simulink model "Modelo_ideal"  (R2021a)
settings: Solver=VariableStepAuto  StartTime=0.0  StopTime=7  RelTol=1e-3
values from neighbouring files (symbols this model uses):
  alpha = 0.5    [Parametros.m]
  Cc = 1000    [Parametros.m]
  Cmax = 900    [Parametros.m]
  Cmin = 100    [Parametros.m]
  Kc = 16000    [Parametros.m]
  Kr = 160000    [Parametros.m]
  Mc = 250    [Parametros.m]
  Mr = 45    [Parametros.m]
undefined symbols (not defined in the file or in its folder): sigbuilder_block
settings Model: Creator=fhlla  LastModifiedBy=fhlla

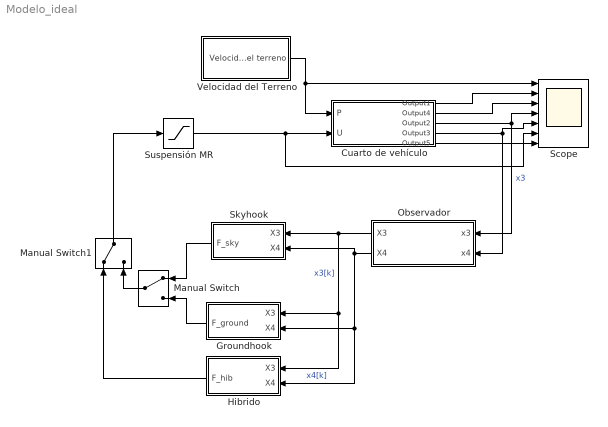
== system Modelo_ideal ==
  Cuarto de vehículo : Subsystem
  Groundhook : Subsystem
  Hibrido : Subsystem
  Manual Switch : ManualSwitch
  Manual Switch1 : ManualSwitch
  Observador : Subsystem
  Scope : Scope  NumInputPorts=7
  Skyhook : Subsystem
  Suspensión MR : Saturate  UpperLimit=10000  LowerLimit=-10000
  Velocidad del Terreno : Subsystem  Tag=STV Subsys  LoadFcn=sigbuilder_block('load');  StartFcn=sigbuilder_block('start');  StopFcn=sigbuilder_block('stop');  ClipboardFcn=sigbuilder_block('clipboard');  mask(Sigbuilder block){tuvar=[0:10]}
      mask help: Simulink:masks:SigbuilderBlock_MD
      mask init:
      | if ~strcmp(get_param(bdroot(gcbh),'SimulationStatus'),'stopped') tuvar = sigbuilder_block('maskInit'); end
      settings: CopyFcn=sigbuilder_block('copy');  DeleteFcn=sigbuilder_block('delete');  ModelCloseFcn=sigbuilder_block('modelClose');  PreSaveFcn=sigbuilder_block('preSave');  PauseFcn=sigbuilder_block('pause');  ContinueFcn=sigbuilder_block('continue');  NameChangeFcn=sigbuilder_block('namechange');  OpenFcn=sigbuilder_block('open',[0 30 1024.5 488.25 ]);  CloseFcn=sigbuilder_block('close');
      mask Display: plot(0, 0, 100, 100,[2, 2, 32, 32, 2], [68, 8, 8, 68, 68],[32, 2], [38, 38], [32, 19, 2],[53, 60, 44], [32, 17, 17, 2],[16, 16, 31, 31]);txt = getActiveGroup(gcbh);text(2, 100, txt,'verticalAlignment', 'top');
  wires:
  Suspensión MR/1 -> Cuarto de vehículo/2(U), Scope/6
  Velocidad del Terreno/1(Velocidad del terreno) -> Cuarto de vehículo/1(P), Scope/1
  Cuarto de vehículo/3(Output2) -> Observador/1(x3), Scope/4  "x3"
  Cuarto de vehículo/4(Output3) -> Observador/2(x4), Scope/5
  Skyhook/1(F_sky) -> Manual Switch/1
  Groundhook/1(F_ground) -> Manual Switch/2
  Cuarto de vehículo/1(Output1) -> Scope/2
  Cuarto de vehículo/2(Output4) -> Scope/3
  Observador/1(X3) -> Skyhook/1(X3), Hibrido/1(X3), Groundhook/1(X3)  "x3[k]"
  Observador/2(X4) -> Skyhook/2(X4), Hibrido/2(X4), Groundhook/2(X4)  "x4[k]"
  Manual Switch1/1 -> Suspensión MR/1
  Manual Switch/1 -> Manual Switch1/2
  Hibrido/1(F_hib) -> Manual Switch1/1
  Cuarto de vehículo/5(Output5) -> Scope/7

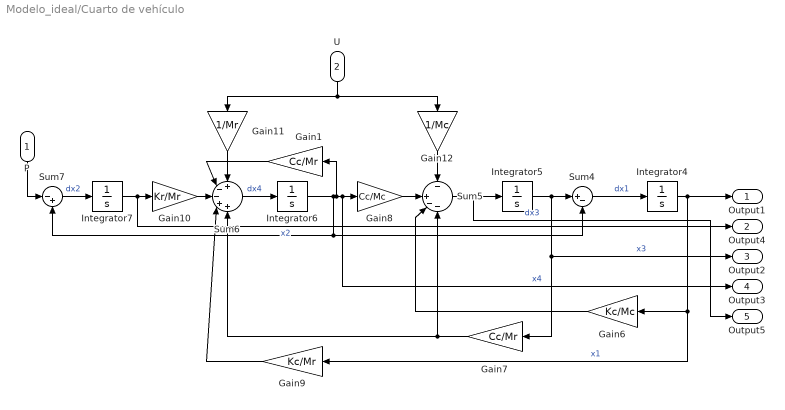
== system Modelo_ideal/Cuarto de vehículo ==
  P : Inport
  U : Inport  Port=2
  Gain1 : Gain  Gain=Cc/Mr
  Gain10 : Gain  Gain=Kr/Mr
  Gain11 : Gain  Gain=1/Mr
  Gain12 : Gain  Gain=1/Mc
  Gain6 : Gain  Gain=Kc/Mc
  Gain7 : Gain  Gain=Cc/Mr
  Gain8 : Gain  Gain=Cc/Mc
  Gain9 : Gain  Gain=Kc/Mr
  Integrator{4..7} (4 alike) : Integrator
  Sum4 : Sum  Inputs=|+-
  Sum5 : Sum  Inputs=-|+--
  Sum6 : Sum  Inputs=+--++
  Sum7 : Sum  Inputs=|-+
  Output1 : Outport
  Output4 : Outport  Port=2
  Output2 : Outport  Port=3
  Output3 : Outport  Port=4
  Output5 : Outport  Port=5
  wires:
  Gain6/1 -> Sum5/3
  Gain11/1 -> Sum6/1
  Gain8/1 -> Sum5/2
  Integrator5/1 -> Sum4/1, Output2/1, Gain7/1  "x3"
  Integrator7/1 -> Output4/1, Gain10/1  "x2"
  Integrator4/1 -> Gain9/1, Gain6/1, Output1/1  "x1"
  Gain10/1 -> Sum6/3
  Sum4/1 -> Integrator4/1  "dx1"
  Gain9/1 -> Sum6/4
  Gain7/1 -> Sum6/5, Sum5/4
  Sum5/1 -> Output5/1, Integrator5/1  "dx3"
  U/1 -> Gain12/1, Gain11/1
  Sum7/1 -> Integrator7/1  "dx2"
  P/1 -> Sum7/1
  Integrator6/1 -> Gain1/1, Output3/1, Gain8/1, Sum7/2, Sum4/2  "x4"
  Gain12/1 -> Sum5/1
  Sum6/1 -> Integrator6/1  "dx4"
  Gain1/1 -> Sum6/2

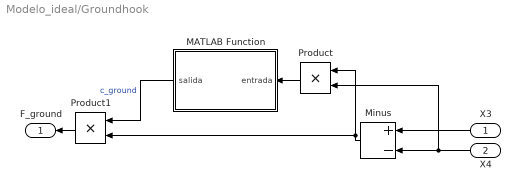
== system Modelo_ideal/Groundhook ==
  X3 : Inport
  X4 : Inport  Port=2
  MATLAB Function : MATLAB Function  TreatAsAtomicUnit=on
  Minus : Sum  Inputs=+-
  Product : Product
  Product1 : Product
  F_ground : Outport
  wires:
  Product/1 -> MATLAB Function/1(entrada)
  X4/1 -> Minus/2, Product/2
  Product1/1 -> F_ground/1
  Minus/1 -> Product1/2, Product/1
  MATLAB Function/1(salida) -> Product1/1  "c_ground"
  X3/1 -> Minus/1

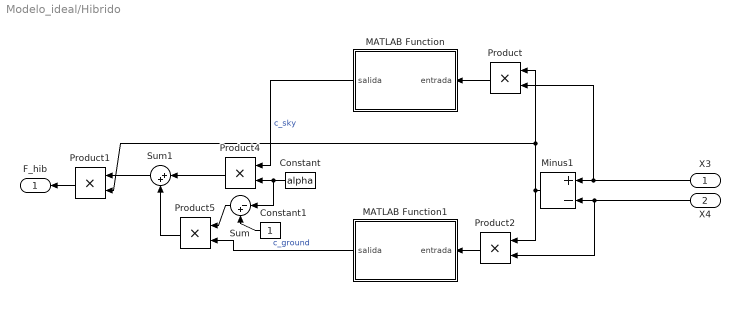
== system Modelo_ideal/Hibrido ==
  X3 : Inport
  X4 : Inport  Port=2
  Constant : Constant  Value=alpha
  Constant1 : Constant
  MATLAB Function : MATLAB Function  TreatAsAtomicUnit=on
  MATLAB Function1 : MATLAB Function  TreatAsAtomicUnit=on
  Minus1 : Sum  Inputs=+-
  Product{,1..2,4..5} (5 alike) : Product
  Sum : Sum  Inputs=|-+
  Sum1 : Sum  Inputs=|++
  F_hib : Outport
  wires:
  Product/1 -> MATLAB Function/1(entrada)
  MATLAB Function/1(salida) -> Product4/1  "c_sky"
  X3/1 -> Product/2, Minus1/1
  X4/1 -> Product2/2, Minus1/2
  Minus1/1 -> Product2/1, Product1/2, Product/1
  Product2/1 -> MATLAB Function1/1(entrada)
  MATLAB Function1/1(salida) -> Product5/2  "c_ground"
  Constant/1 -> Sum/1, Product4/2
  Constant1/1 -> Sum/2
  Sum/1 -> Product5/1
  Product5/1 -> Sum1/2
  Product4/1 -> Sum1/1
  Sum1/1 -> Product1/1
  Product1/1 -> F_hib/1

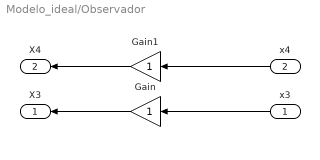
== system Modelo_ideal/Observador ==
  x3 : Inport
  x4 : Inport  Port=2
  Gain : Gain
  Gain1 : Gain
  X3 : Outport
  X4 : Outport  Port=2
  wires:
  x3/1 -> Gain/1
  x4/1 -> Gain1/1
  Gain/1 -> X3/1
  Gain1/1 -> X4/1

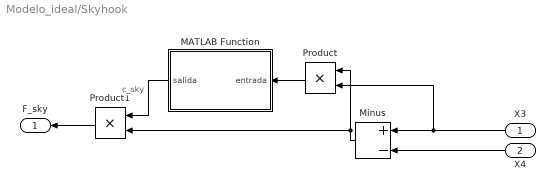
== system Modelo_ideal/Skyhook ==
  X3 : Inport
  X4 : Inport  Port=2
  MATLAB Function : MATLAB Function  TreatAsAtomicUnit=on
  Minus : Sum  Inputs=+-
  Product : Product
  Product1 : Product
  F_sky : Outport
  wires:
  Minus/1 -> Product1/2, Product/1
  Product/1 -> MATLAB Function/1(entrada)
  MATLAB Function/1(salida) -> Product1/1  "c_sky"
  Product1/1 -> F_sky/1
  X4/1 -> Minus/2
  X3/1 -> Product/2, Minus/1

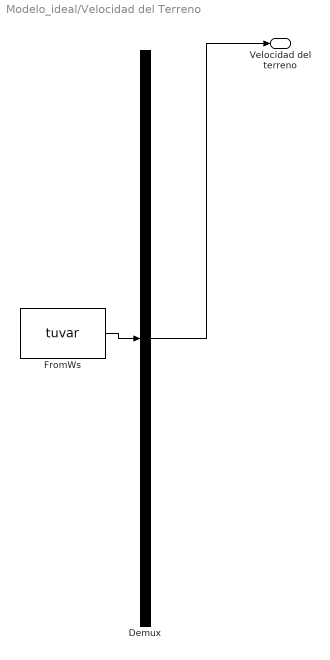
== system Modelo_ideal/Velocidad del Terreno ==
  Demux : Demux  Tag=STV Demux  Outputs=1
  FromWs : FromWorkspace  Tag=STV FromWs  VariableName=tuvar  SampleTime=0
      SigBuilderData=|
      | common.afterFinalStr = 'Extrapolate'
      | common.sampleTime = 0
      | dataSet.timeRange = [0 11.5]
      | dataSet.name = 'Group 1'
      | sbobj.Groups.Name = 'Group 1'
      | sbobj.Groups.Signals.Name = 'Velocidad del terreno'
      | sbobj.Groups.Signals.XData = [0 1 1 1.0034 1.0034 1.0068 1.0068 1.0102 1.0102 11.5]
      | sbobj.Groups.Signals.YData = [0 0 14.71 14.71 0 0 -14.71 -14.71 0 0]
      | sbobj.Groups.TimeRange = [0 11.5]
  Velocidad del terreno : Outport  Tag=STV Outport
  wires:
  FromWs/1 -> Demux/1
  Demux/1 -> Velocidad del terreno/1

== matlab function Modelo_ideal/Groundhook/MATLAB Function ==
  data: entrada input; salida output; Cmax parameter; Cmin parameter
function salida = groundhook(entrada, Cmax, Cmin)
    if entrada<=0
        salida = Cmax % c_ground_max;
    else
        salida = Cmin % c_ground_min;
    end
end

== matlab function Modelo_ideal/Skyhook/MATLAB Function ==
  data: entrada input; salida output; Cmax parameter; Cmin parameter
function salida = skyhook(entrada, Cmax, Cmin)
    if entrada>=0
        salida = Cmax % c_sky_max;
    else
        salida = Cmin % c_sky_min;   200
    end
end

== matlab function Modelo_ideal/Hibrido/MATLAB Function ==
  data: entrada input; salida output; Cmax parameter; Cmin parameter
function salida = skyhook(entrada, Cmax, Cmin)
    if entrada>=0
        salida = Cmax % c_sky_max;
    else
        salida = Cmin % c_sky_min;   200
    end
end

== matlab function Modelo_ideal/Hibrido/MATLAB Function1 ==
  data: entrada input; salida output; Cmax parameter; Cmin parameter
function salida = groundhook(entrada, Cmax, Cmin)
    if entrada<=0
        salida = Cmax % c_ground_max;
    else
        salida = Cmin % c_ground_min;
    end
end
